simulink model "adc_test"  (R2023b)
settings: Solver=VariableStepAuto  StartTime=0.0  StopTime=100  RelTol=1e-3
libraries: canmsglib x1, c280xlib x1, c2802xlib x1
settings Model: Creator=Columbia  LastModifiedBy=Columbia

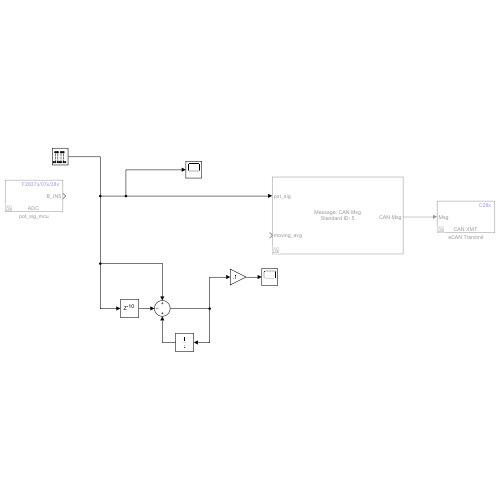
[thumbnail: Simulink's stored preview of the top-level diagram]
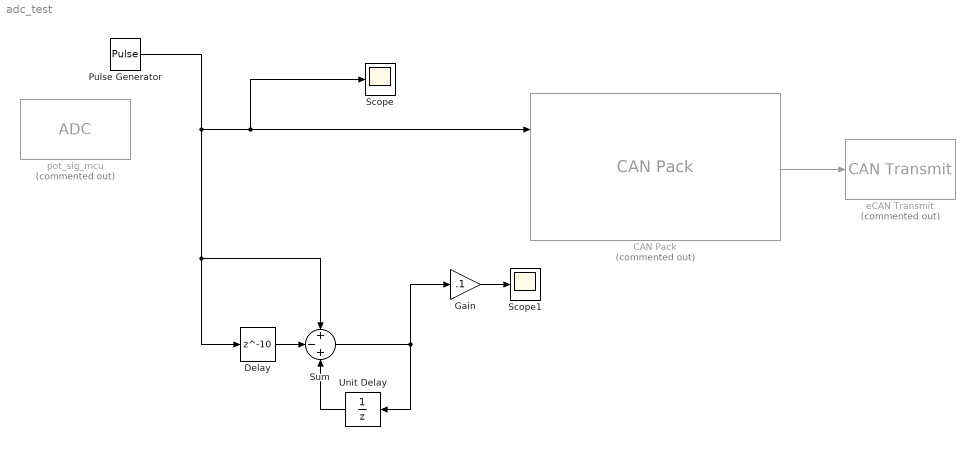
== system adc_test ==
  CAN Pack : canmsglib/CAN Pack  Commented=on  MsgList=(none)  MsgName=CAN Msg  MsgIDType=Standard (11-bit identifier)  MsgIdentifier=5  MsgLength=8  Remote=off  ApplyMinMax=off  BusOutput=off  SignalInfo={ 'pot_sig', '0', '8', 'LE', 'unsigned', 'Standard', '0', '1', '0', '-Inf', 'Inf'; 'moving_avg', '8', '8', 'LE', 'signed', 'Standard', '0', '1', '0', '-Inf', 'Inf' }
      settings: DataFormat=manually specified signals
  Delay : Delay  DelayLength=10
  Gain : Gain  Gain=.1
  Pulse Generator : DiscretePulseGenerator  Period=20  PulseWidth=3
  Scope : Scope
  Scope1 : Scope
  Sum : Sum  Inputs=+-+
  Unit Delay : UnitDelay  SampleTime=-1  HasFrameUpgradeWarning=on
  eCAN Transmit : c280xlib/CAN Transmit  Commented=on  chipFamily=C280x  useModule=CAN_B  mailboxNo=5  messageID=5  messageType=Standard (11-bit identifier)  enableBlockingMode=off  postInterrupt=off  interruptLine=0
  pot_sig_mcu : c2802xlib/ADC  Commented=on  blkParamProc=C2000_Type4  ADCModule=B  samplingMode=Single sample mode  ADCResolution=12-bit (Single-ended input)  useSOC1=SOC6  useSOC2=SOC0_SOC1  SOCAcquisitionWindow=60  SOCTriggerSource=Software  SOCInterruptTrigger=No ADCINT  Ts=0.001  dType=uint16  postInterrupt=off  interruptSel=ADCINT1  ADCINTContinuous=on  endma=off  chdma=1  conv1=ADCINA0  conv2=ADCINA0 and ADCINB0  conv1_Type4=ADCIN5  conv2_Type4=ADCIN0 and ADCIN1
  wires:
  Pulse Generator/1 -> CAN Pack/1, Scope/1, Delay/1, Sum/1
  CAN Pack/1 -> eCAN Transmit/1
  Unit Delay/1 -> Sum/3
  Delay/1 -> Sum/2
  Sum/1 -> Gain/1, Unit Delay/1
  Gain/1 -> Scope1/1
